simulink model "Mod_simplepend_R2018A"  (R2018b)
settings: Solver=VariableStepAuto  StartTime=0.0  StopTime=60  RelTol=1e-3
undefined symbols (not defined in the file or in its folder): par
settings Model: Creator=janneke  LastModifiedBy=janneke

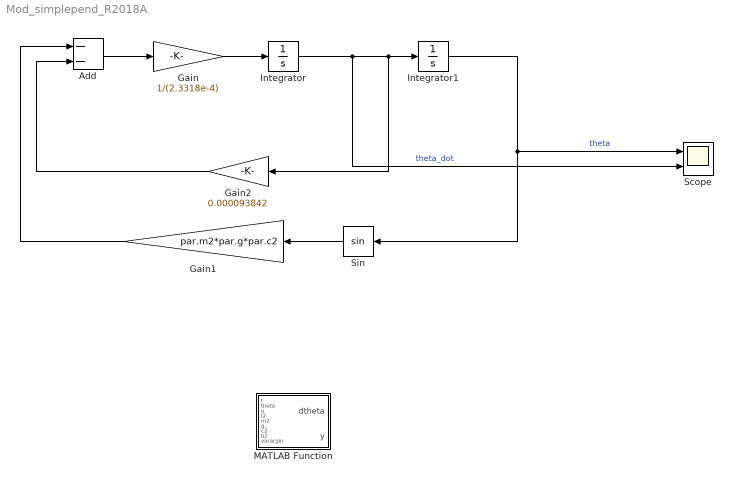
== system Mod_simplepend_R2018A ==
  Add : Sum  Inputs=--
  Gain : Gain  Gain=1/(2.3318e-4)
  Gain1 : Gain  Gain=par.m2*par.g*par.c2
  Gain2 : Gain  Gain=0.000093842
  Integrator : Integrator
  Integrator1 : Integrator  InitialCondition=-pi/2
  MATLAB Function : MATLAB Function  TreatAsAtomicUnit=on
  Scope : Scope  NumInputPorts=2
  Sin : Trigonometry
  wires:
  Integrator/1 -> Scope/2, Gain2/1, Integrator1/1  "theta_dot"
  Integrator1/1 -> Sin/1, Scope/1  "theta"
  Gain/1 -> Integrator/1
  Add/1 -> Gain/1
  Sin/1 -> Gain1/1
  Gain1/1 -> Add/1
  Gain2/1 -> Add/2

== matlab function Mod_simplepend_R2018A/MATLAB Function ==
  data: t input; theta input; dtheta output; u input; y output; I2 input; m2 input; g input; c2 input; b2 input; varargin input
function [dtheta,y] = nonlinmod(t,theta,u,I2,m2,g,c2,b2,varargin)

dtheta(1) = theta(2);
dtheta(2) = 1/I2*(-m2*g*c2*sin(theta(1))-b2*theta(2));

y = theta(1);
end
